simulink model "Test_of_Wave_Suction_Force_Observer_in_Finite_Time_tau_w"  (R2023a)
settings: Solver=FixedStepAuto  StartTime=0.0  StopTime=150  FixedStep=1e-3  RelTol=1e-3
libraries: simulink x2
settings Model: Creator=邓宇飞  LastModifiedBy=邓宇飞

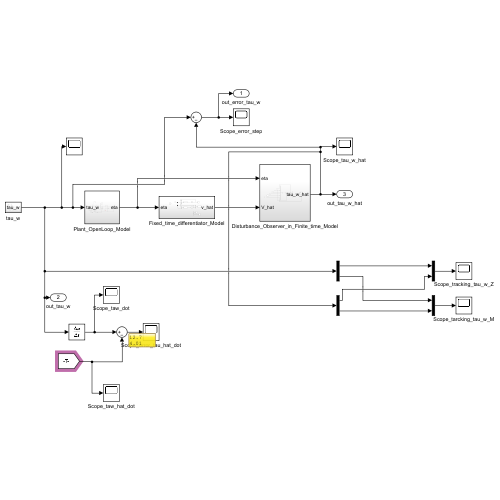
[thumbnail: Simulink's stored preview of the top-level diagram]
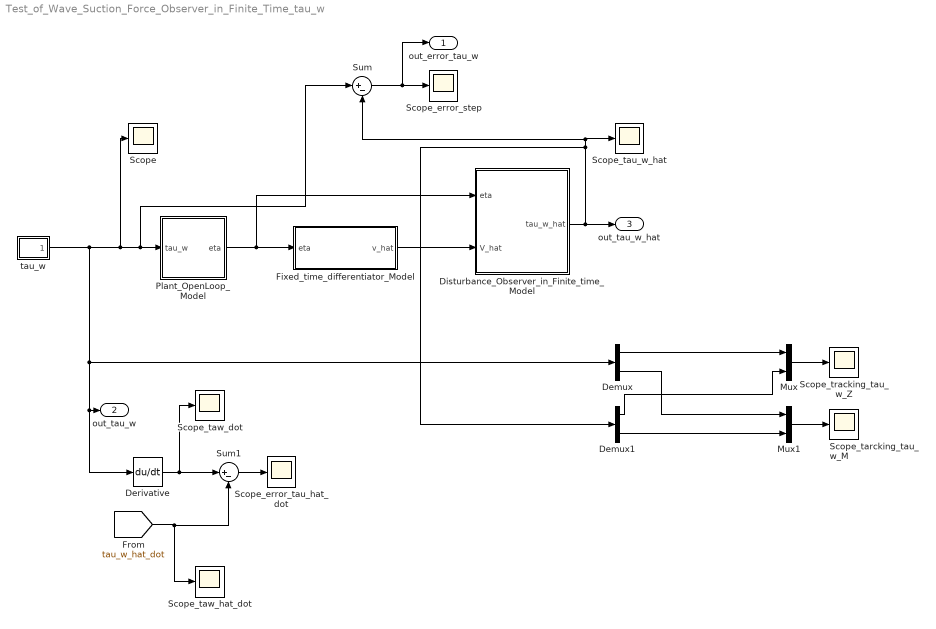
== system Test_of_Wave_Suction_Force_Observer_in_Finite_Time_tau_w ==
  Demux : Demux  Outputs=2
  Demux1 : Demux  Outputs=2
  Derivative : Derivative
  Disturbance_Observer_in_Finite_time_Model : Subsystem
  Fixed_time_differentiator_Model : Subsystem
  Mux : Mux  Inputs=2
  Mux1 : Mux  Inputs=2
  Plant_OpenLoop_Model : Subsystem
  Scope : Scope
  Scope_error_step : Scope
  Scope_error_tau_hat_dot : Scope
  Scope_tarcking_tau_w_M : Scope
  Scope_tau_w_hat : Scope
  Scope_taw_dot : Scope
  Scope_taw_hat_dot : Scope
  Scope_tracking_tau_w_Z : Scope
  Sum : Sum  Inputs=|+-
  Sum1 : Sum  Inputs=|+-
  tau_w : Subsystem
  out_error_tau_w : Outport
  out_tau_w : Outport  Port=2
  out_tau_w_hat : Outport  Port=3
  wires:
  Fixed_time_differentiator_Model/1(v_hat) -> Disturbance_Observer_in_Finite_time_Model/2(V_hat)
  tau_w/1(tau_w) -> Demux/1, Derivative/1, out_tau_w/1, Scope/1, Sum/1, Plant_OpenLoop_Model/1(tau_w)
  Sum/1 -> out_error_tau_w/1, Scope_error_step/1
  Disturbance_Observer_in_Finite_time_Model/1(tau_w_hat) -> Sum/2, Scope_tau_w_hat/1, Demux1/1, out_tau_w_hat/1
  Plant_OpenLoop_Model/1(eta) -> Disturbance_Observer_in_Finite_time_Model/1(eta), Fixed_time_differentiator_Model/1(eta)
  Mux/1 -> Scope_tracking_tau_w_Z/1
  Mux1/1 -> Scope_tarcking_tau_w_M/1
  Demux/1 -> Mux/1
  Demux1/1 -> Mux/2
  Demux/2 -> Mux1/1
  Demux1/2 -> Mux1/2
  Derivative/1 -> Scope_taw_dot/1, Sum1/1
  [tau_w_hat_dot] -> Sum1/2, Scope_taw_hat_dot/1
  Sum1/1 -> Scope_error_tau_hat_dot/1

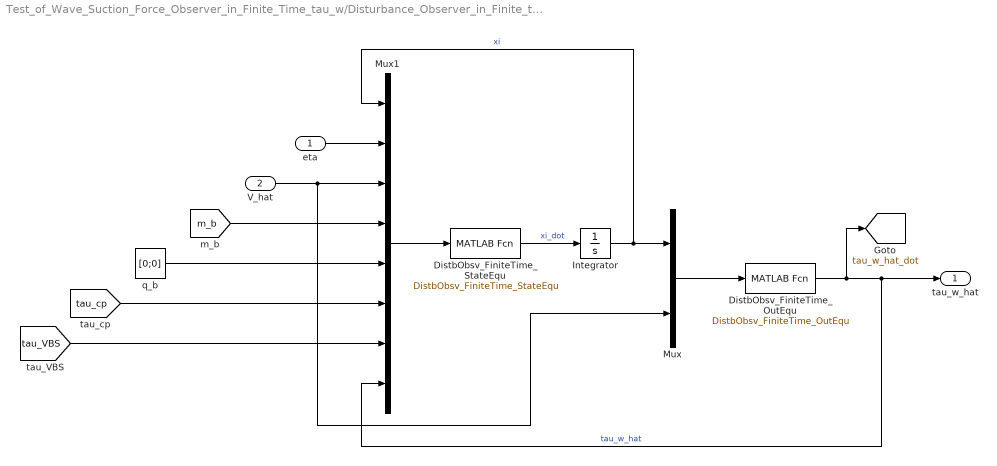
== system Test_of_Wave_Suction_Force_Observer_in_Finite_Time_tau_w/Disturbance_Observer_in_Finite_time_Model ==
  eta : Inport  PortDimensions=2
  V_hat : Inport  Port=2  PortDimensions=2
  DistbObsv_FiniteTime_OutEqu : MATLABFcn  MATLABFcn=DistbObsv_FiniteTime_OutEqu  OutputDimensions=2
  DistbObsv_FiniteTime_StateEqu : MATLABFcn  MATLABFcn=DistbObsv_FiniteTime_StateEqu  OutputDimensions=2
  Integrator : Integrator
  Mux : Mux  Inputs=2
  Mux1 : Mux  Inputs=8
  q_b : Constant  Value=[0;0]
  tau_w_hat : Outport
  tag scope: tau_w_hat_dot=global
  wires:
  Mux1/1 -> DistbObsv_FiniteTime_StateEqu/1
  q_b/1 -> Mux1/5
  [tau_cp] -> Mux1/6
  V_hat/1 -> Mux/2, Mux1/3
  [tau_VBS] -> Mux1/7
  DistbObsv_FiniteTime_OutEqu/1 -> [tau_w_hat_dot], tau_w_hat/1, Mux1/8  "tau_w_hat"
  Integrator/1 -> Mux1/1, Mux/1  "xi"
  Mux/1 -> DistbObsv_FiniteTime_OutEqu/1
  DistbObsv_FiniteTime_StateEqu/1 -> Integrator/1  "xi_dot"
  eta/1 -> Mux1/2
  [m_b] -> Mux1/4

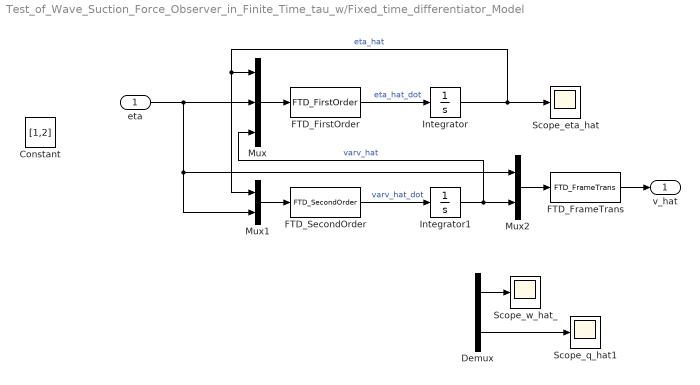
== system Test_of_Wave_Suction_Force_Observer_in_Finite_Time_tau_w/Fixed_time_differentiator_Model ==
  eta : Inport
  Constant : Constant  Value=[1,2]
  Demux : Demux  Outputs=2
  FTD_FirstOrder : MATLABFcn  MATLABFcn=FTD_FirstOrder  OutputDimensions=2
  FTD_FrameTrans : MATLABFcn  MATLABFcn=FTD_FrameTrans
  FTD_SecondOrder : MATLABFcn  MATLABFcn=FTD_SecondOrder  OutputDimensions=2
  Integrator : Integrator
  Integrator1 : Integrator
  Mux : Mux  Inputs=3
  Mux1 : Mux  Inputs=2
  Mux2 : Mux  Inputs=2
  Scope_eta_hat : Scope
  Scope_q_hat1 : Scope
  Scope_w_hat_ : Scope
  v_hat : Outport
  wires:
  Demux/1 -> Scope_w_hat_/1
  Integrator/1 -> Mux1/1, Mux/1, Scope_eta_hat/1  "eta_hat"
  Integrator1/1 -> Mux/3, Mux2/2  "varv_hat"
  Mux2/1 -> FTD_FrameTrans/1
  Mux/1 -> FTD_FirstOrder/1
  Mux1/1 -> FTD_SecondOrder/1
  Demux/2 -> Scope_q_hat1/1
  FTD_SecondOrder/1 -> Integrator1/1  "varv_hat_dot"
  FTD_FirstOrder/1 -> Integrator/1  "eta_hat_dot"
  eta/1 -> Mux2/1, Mux1/2, Mux/2
  FTD_FrameTrans/1 -> v_hat/1

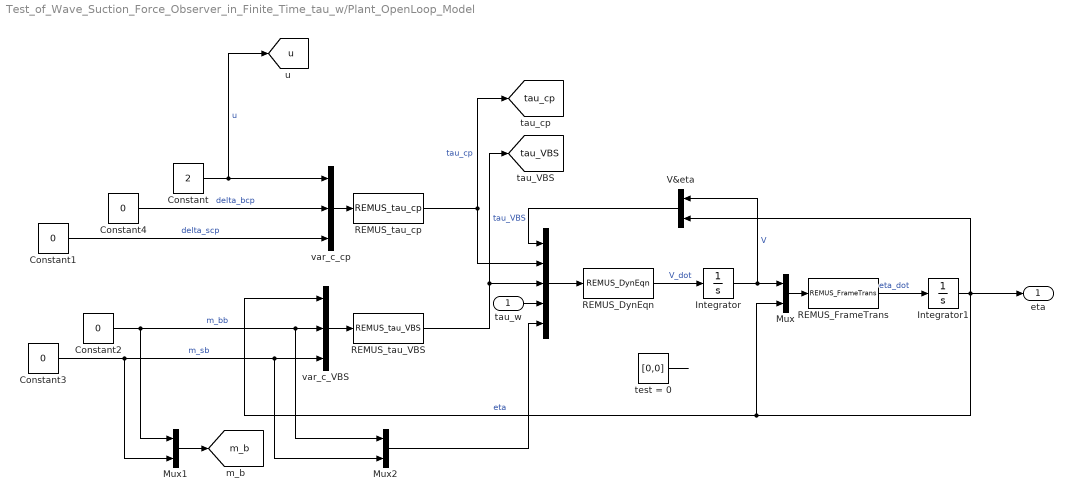
== system Test_of_Wave_Suction_Force_Observer_in_Finite_Time_tau_w/Plant_OpenLoop_Model ==
  tau_w : Inport
  " " : Mux  Inputs=5
  Constant : Constant  Value=2
  Constant{1..4} (4 alike) : Constant  Value=0
  Integrator : Integrator
  Integrator1 : Integrator
  Mux : Mux  Inputs=2
  Mux1 : Mux  Inputs=2
  Mux2 : Mux  Inputs=2
  REMUS_DynEqn : MATLABFcn  MATLABFcn=REMUS_DynEqn  OutputDimensions=2
  REMUS_FrameTrans : MATLABFcn  MATLABFcn=REMUS_FrameTrans  OutputDimensions=2
  REMUS_tau_VBS : MATLABFcn  MATLABFcn=REMUS_tau_VBS  OutputDimensions=2
  REMUS_tau_cp : MATLABFcn  MATLABFcn=REMUS_tau_cp  OutputDimensions=2
  V&eta : Mux  Inputs=2
  test = 0 : Constant  Value=[0,0]
  var_c_VBS : Mux  Inputs=3
  var_c_cp : Mux  Inputs=3
  eta : Outport
  tag scope: m_b=global, tau_VBS=global, tau_cp=global, u=global
  wires:
  Constant/1 -> [u], var_c_cp/1  "u"
  REMUS_DynEqn/1 -> Integrator/1  "V_dot"
  REMUS_tau_cp/1 -> [tau_cp], " "/2  "tau_cp"
  Integrator1/1 -> eta/1, Mux/2, var_c_VBS/1, V&eta/2  "eta"
  Constant1/1 -> var_c_cp/3  "delta_scp"
  test = 0/1 -> ?
  Constant3/1 -> Mux1/2, Mux2/2, var_c_VBS/3  "m_sb"
  Mux/1 -> REMUS_FrameTrans/1
  " "/1 -> REMUS_DynEqn/1
  Integrator/1 -> Mux/1, V&eta/1  "V"
  Constant2/1 -> Mux1/1, Mux2/1, var_c_VBS/2  "m_bb"
  Constant4/1 -> var_c_cp/2  "delta_bcp"
  var_c_cp/1 -> REMUS_tau_cp/1
  V&eta/1 -> " "/1
  REMUS_tau_VBS/1 -> [tau_VBS], " "/3  "tau_VBS"
  tau_w/1 -> " "/4
  REMUS_FrameTrans/1 -> Integrator1/1  "eta_dot"
  var_c_VBS/1 -> REMUS_tau_VBS/1
  Mux1/1 -> [m_b]
  Mux2/1 -> " "/5

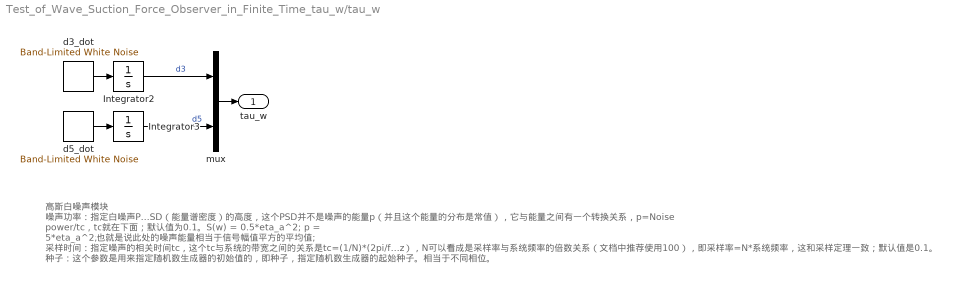
== system Test_of_Wave_Suction_Force_Observer_in_Finite_Time_tau_w/tau_w ==
  note: 高斯白噪声模块
      | 噪声功率：指定白噪声PSD（能量谱密度）的高度，这个PSD并不是噪声的能量p（并且这个能量的分布是常值），它与能量之间有一个转换关系，p=Noise power/tc，tc就在下面；默认值为0.1。S(w) = 0.5*eta_a^2;
      | p = 5*eta_a^2;也就是说此处的噪声能量相当于信号幅值平方的平均值;
      | 采样时间：指定噪声的相关时间tc，这个tc与系统的带宽之间的关系是tc=(1/N)*(2pi/fmax)，其中fmax是系统的带宽（实际上是角频率，fmax=2*pi*f，这个f才是我们常使用的频率Hz），N可以看成是采样率与系统频率的倍数关系（文档中推荐使用100），即采样率=N*系统频率，这和采样定理一致；默认值是0.1。
      | 种子：这个参数是用来指定随机数生成器的初始值的，即种子，指定随机数生成器的起始种子。相当于不同相位。
  Integrator2 : Integrator
  Integrator3 : Integrator
  d3_dot : simulink/Sources/Band-Limited White Noise  Cov=[0.5]  Ts=0.1  seed=[2]
  d5_dot : simulink/Sources/Band-Limited White Noise  Cov=[0.1]  Ts=0.1  seed=[3]
  mux : Mux  Inputs=2
  tau_w : Outport
  wires:
  Integrator3/1 -> mux/2  "d5"
  d5_dot/1 -> Integrator3/1
  d3_dot/1 -> Integrator2/1
  mux/1 -> tau_w/1
  Integrator2/1 -> mux/1  "d3"
